simulink model "Tutorial2_SolarTracker"  (R2020a)
settings: Solver=VariableStepAuto  StartTime=0.0  StopTime=15*3600  RelTol=1e-3
values from neighbouring files (symbols this model uses):
  J = 8.6    [Tutorial2_SolarTracker_Parameters.m]
  K_d = 5    [Tutorial2_SolarTracker_Parameters.m]
  K_f = 1    [Tutorial2_SolarTracker_Parameters.m]
  K_g = 1    [Tutorial2_SolarTracker_Parameters.m]
  K_t = 1    [Tutorial2_SolarTracker_Parameters.m]
  L = 1    [Tutorial2_SolarTracker_Parameters.m]
  R = 1    [Tutorial2_SolarTracker_Parameters.m]
libraries: simulink x1
settings Model: Creator=Dell  LastModifiedBy=Dell
settings DataIOCC: ExternalInput=[sunTime, sunPosition]  LoadExternalInput=on

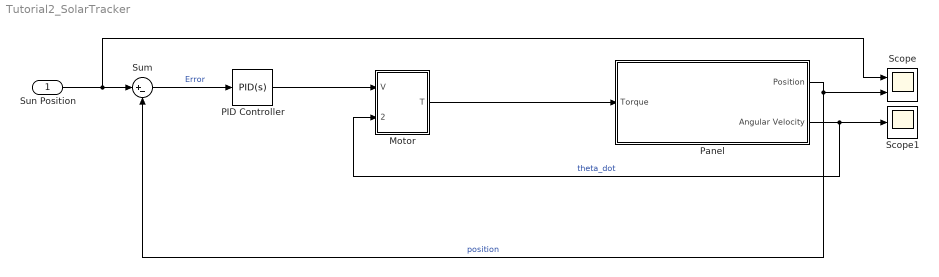
== system Tutorial2_SolarTracker ==
  Sun Position : Inport
  Motor : Subsystem
  PID Controller : simulink/Continuous/PID Controller  Controller=PID  Form=Parallel  TimeDomain=Continuous-time  UseExternalTs=off  SampleTime=-1  IntegratorMethod=Forward Euler  FilterMethod=Forward Euler  ControllerParametersSource=internal  P=8  I=0  D=25  UseFilter=on  N=100  TunerSelectOption=Transfer Function Based (PID Tuner App)  InitialConditionSource=internal  InitialConditionForIntegrator=0  InitialConditionForFilter=0  DifferentiatorICPrevScaledInput=0  ExternalReset=none  TrackingMode=off  Kt=1  LimitOutput=off  UpperSaturationLimit=inf  LowerSaturationLimit=-inf  LinearizeAsGain=on  AntiWindupMode=none  Kb=1  POutMin=[]  POutMax=[]  IOutMin=[]  IOutMax=[]  DOutMin=[]  DOutMax=[]  NOutMin=[]  NOutMax=[]  SumOutMin=[]  SumOutMax=[]  SaturationOutMin=[]  SaturationOutMax=[]  PParamMin=[]  PParamMax=[]  IParamMin=[]  IParamMax=[]  DParamMin=[]  DParamMax=[]  NParamMin=[]  NParamMax=[]  KbParamMin=[]  KbParamMax=[]  KtParamMin=[]  KtParamMax=[]  KbOutMin=[]  KbOutMax=[]  KtOutMin=[]  KtOutMax=[]  IntegratorOutMin=[]  IntegratorOutMax=[]  FilterOutMin=[]  FilterOutMax=[]  SumI1OutMin=[]  SumI1OutMax=[]  SumI2OutMin=[]  SumI2OutMax=[]  SumI3OutMin=[]  SumI3OutMax=[]  SumI4OutMin=[]  SumI4OutMax=[]  SumDOutMin=[]  SumDOutMax=[]  DifferentiatorOutMin=[]  DifferentiatorOutMax=[]  FilterDiffOutCoefMin=[]  FilterDiffOutCoefMax=[]  ReciprocalOutMin=[]  ReciprocalOutMax=[]  SumDenOutMin=[]  SumDenOutMax=[]  SumNumOutMin=[]  SumNumOutMax=[]  DivideOutMin=[]  DivideOutMax=[]  UdiffTsProdOutMin=[]  UdiffTsProdOutMax=[]  NTsProdOutMin=[]  NTsProdOutMax=[]  UintegralTsProdOutMin=[]  UintegralTsProdOutMax=[]  UngainTsProdOutMin=[]  UngainTsProdOutMax=[]  IntegratorContinuousStateAttributes=''  IntegratorStateMustResolveToSignalObject=off  IntegratorRTWStateStorageClass=Auto  FilterContinuousStateAttributes=''  FilterStateMustResolveToSignalObject=off  FilterRTWStateStorageClass=Auto  ParallelPVariant=InternalParameters  IdealPVariant=Disabled  IVariant=InternalParameters  DVariant=InternalParameters  IntegratorVariant=Continuous  SatVariant=Disabled  AWVariant=Passthrough  PCopyVariant=Disabled  TRVariant=Disabled  FdbkBlocksVariant=Forward  IdealPFdbkVariant=Disabled  SatFdbkVariant=Disabled  DerivativeFilterVariant=ContFilter  NVariant=InternalParameters  NCopyVariant=Disabled  FilterICVariant=InternalICsFilter  IntegratorICVariant=InternalICs  ExternalResetVariant=Disabled  TRSumVariant=Passthrough  SumFdbkVariant=Disabled  SumVariant=Sum_PID  TsampFilterVariant=InternalTs  TsampNgainVariant=Passthrough  TsampIntegralVariant=Passthrough
  Panel : Subsystem
  Scope : Scope  NumInputPorts=2
  Scope1 : Scope
  Sum : Sum  Inputs=|+-
  wires:
  Panel/1(Position) -> Scope/2, Sum/2  "position"
  Panel/2(Angular Velocity) -> Motor/2(theta_dot), Scope1/1  "theta_dot"
  Sum/1 -> PID Controller/1  "Error"
  Motor/1(T) -> Panel/1(Torque)
  Sun Position/1 -> Scope/1, Sum/1
  PID Controller/1 -> Motor/1(V)

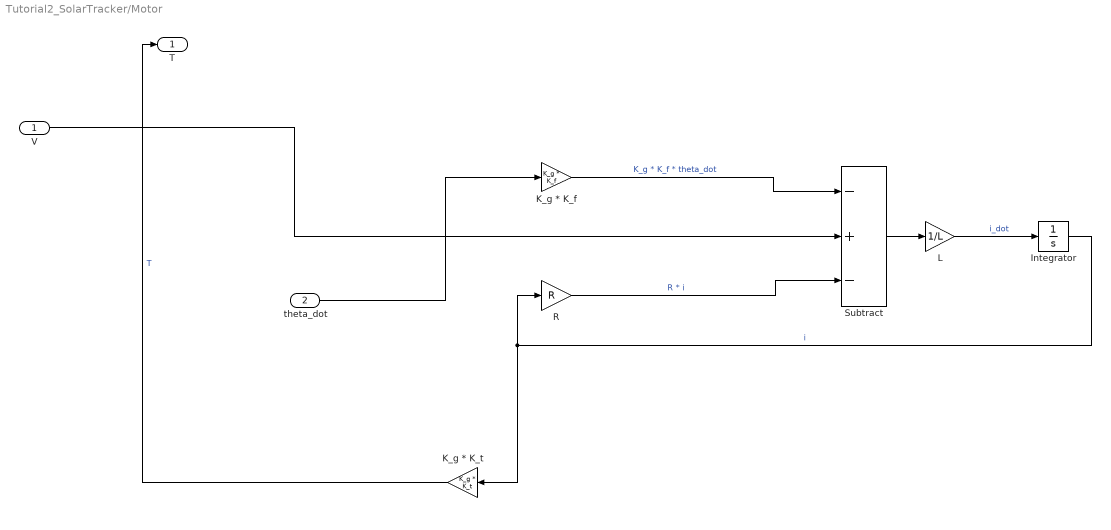
== system Tutorial2_SolarTracker/Motor ==
  V : Inport
  theta_dot : Inport  Port=2
  Integrator : Integrator
  K_g * K_f : Gain  Gain=K_g * K_f
  K_g * K_t : Gain  Gain=K_g * K_t
  L : Gain  Gain=1/L
  R : Gain  Gain=R
  Subtract : Sum  Inputs=-+-
  T : Outport
  wires:
  Integrator/1 -> K_g * K_t/1, R/1  "i"
  K_g * K_f/1 -> Subtract/1  "K_g * K_f * theta_dot"
  R/1 -> Subtract/3  "R * i"
  L/1 -> Integrator/1  "i_dot"
  K_g * K_t/1 -> T/1  "T"
  Subtract/1 -> L/1
  theta_dot/1 -> K_g * K_f/1
  V/1 -> Subtract/2

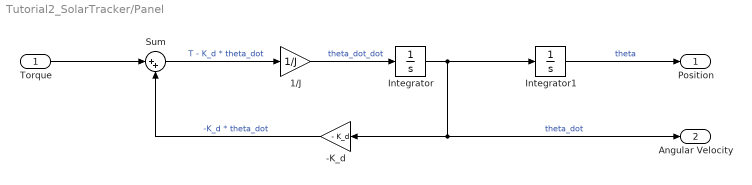
== system Tutorial2_SolarTracker/Panel ==
  Torque : Inport
  -K_d : Gain  Gain=- K_d
  1/J : Gain  Gain=1/J
  Integrator : Integrator
  Integrator1 : Integrator
  Sum : Sum  Inputs=|++
  Position : Outport
  Angular Velocity : Outport  Port=2
  wires:
  1/J/1 -> Integrator/1  "theta_dot_dot"
  Integrator/1 -> Angular Velocity/1, -K_d/1, Integrator1/1  "theta_dot"
  -K_d/1 -> Sum/2  "-K_d * theta_dot"
  Torque/1 -> Sum/1
  Sum/1 -> 1/J/1  "T - K_d * theta_dot"
  Integrator1/1 -> Position/1  "theta"
